simulink model "Simulinkquestao1"  (R2020a)
settings: Solver=FixedStepAuto  StartTime=0.0  StopTime=10.0  FixedStep=1e-3  RelTol=1e-3
settings Model: Creator=Dylan  LastModifiedBy=Dylan

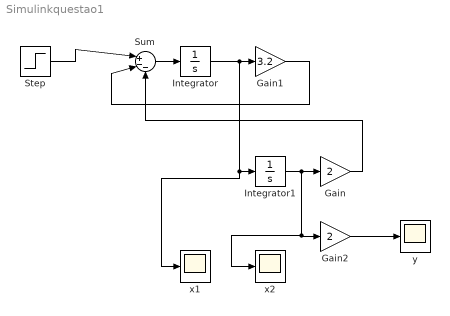
== system Simulinkquestao1 ==
  Gain : Gain  Gain=2
  Gain1 : Gain  Gain=3.2
  Gain2 : Gain  Gain=2
  Integrator : Integrator
  Integrator1 : Integrator
  Step : Step  Time=0  OutDataTypeStr=single  SampleTime=0
  Sum : Sum  Inputs=|+--
  x1 : Scope
  x2 : Scope
  y : Scope
  wires:
  Sum/1 -> Integrator/1
  Integrator/1 -> x1/1, Integrator1/1, Gain1/1
  Gain1/1 -> Sum/2
  Integrator1/1 -> x2/1, Gain2/1, Gain/1
  Gain/1 -> Sum/3
  Gain2/1 -> y/1
  Step/1 -> Sum/1
